simulink library "rappid_564xl_ec_toolbox"  (Simulink 8.1)
settings: Solver=FixedStepDiscrete  StartTime=0.0  StopTime=10.0  RelTol=1e-3
undefined symbols (not defined in the file or in its folder): CTU_unit, mem_AddrLW, mem_AddrUP, rappid_564xl_adc_input_support_rev2, rappid_564xl_can_support_rev2, read_mem_AddrLW, read_mem_AddrUP
(part 1 of 5)
settings Model: Creator=r61406  LastModifiedBy=evarshavskaya

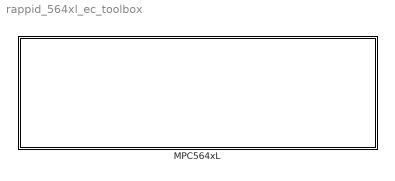
== system rappid_564xl_ec_toolbox ==
  MPC564xL : Subsystem

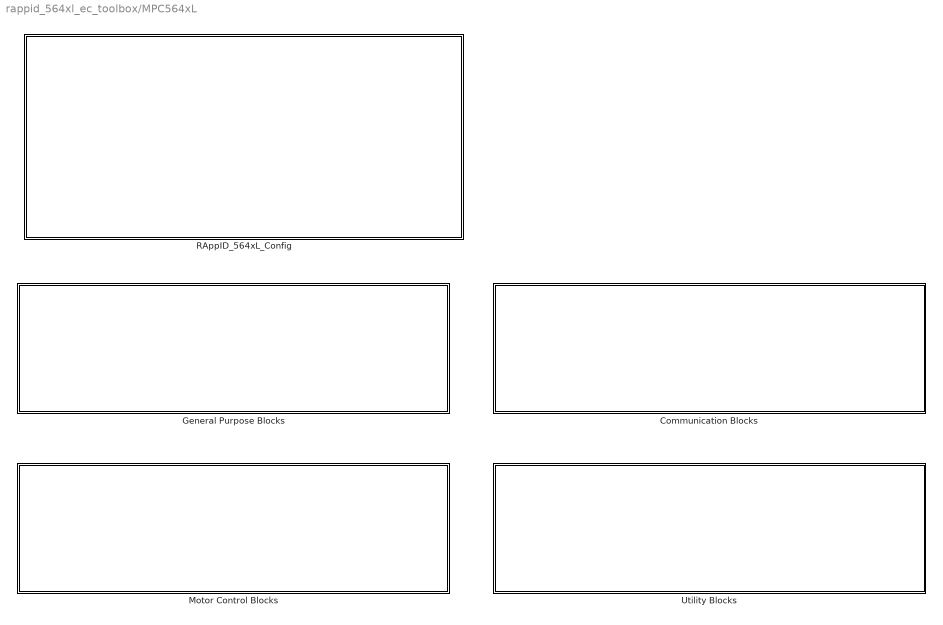
== system rappid_564xl_ec_toolbox/MPC564xL ==
  Communication Blocks : Subsystem
  General Purpose Blocks : Subsystem
  Motor Control Blocks : Subsystem
  RAppID_564xL_Config : Subsystem  LoadFcn=|  InitFcn=|  mask(RAppID_EC_564xL){SystemClock=120, XTAL=40, MC_clock_60=12, MC_clock_80=16, MC_clock_120=10, SWG_clock_60=20, SWG_clock_80=13.334, SWG_clock_120=20, Compiler=CodeWarrior, MemTarget=RAM, Part=MPC5643L, Package=144 LQFP, global_int_priority=11, base_tick_priority=12, sys_task_supress=off, exception_handlers=off, stored_mdl_name=can_simple_block__, freemaster_interface=Oops, freemaster_rx_pin=LINFlex_0 Rx Pin 116 : "PB[3]", freemaster_tx_pin=LINFlex_0 Tx Pin 114 : "PB[2]", freemaster_interface_1=None, freemaster_enable=off, freemaster_rate=57600, freemaster_tx0_pin=18 : B[2] : 114 : A14, freemaster_rx0_pin=19 : B[3] : 116 : B13, freemaster_tx1_pin=57 : D[9] : 26 : L3, freemaster_rx1_pin=29 : B[13] : 60 : R10, freemaster_can_channel=1CH, freemater_can_speed=500K, freemaster_can_msgig=0x7AA, ccp_interface=None, ccp_enable=off, ccp_can_channel=CH1 (MB 0 - 1), ccp_can_speed=500K, ccp_can_cro_id=256, ccp_can_dto_id=257, ccp_dev_id=RappID, ccp_dev_addr=0, ccp_odt=3, ccp_daq=3, pil_enable=off, pil_bam=off, comport=1, pil_rate=57600, bam_password_def=on, bam_password=0xFEEDFACECAFEBEEF, bam_sa_cs=off, bam_start_address=0x0, bam_code_size=0x7000, cons_dspi=on, cons_can=on, cons_adc=on, cons_pwm=on, cons_ctu=on, cons_swg=on, cons_eTimer=on, cons_fm=on}
      | rappid_564xl_set_cur_model(bdroot(gcs));
      | rappid_564xl_block_load(bdroot(gcs)); 
      | rappid_564xl_fmaster_config(gcb);
      | rappid_564xl_set_cur_model(bdroot(gcs));
      | rappid_564xl_update_model('init');
      | rappid_564xl_check('RAppID_EC_564xL');
      | rappid_564xl_consistency_checks( bdroot(gcs));
      mask prompts: SystemClock "Select System Clock Mhz"; XTAL "Select External Crystal Value Mhz"; MC_clock_60 "Motor control clock, MHz  (3.75 - 60)"; MC_clock_80 "Motor control clock, MHz  (5 - 80)"; MC_clock_120 "Motor control clock, MHz  (7.5 - 120)"; SWG_clock_60 "SWG clock, MHz  (12 - 20)"; SWG_clock_80 "SWG clock, MHz  (13.334 - 20)"; SWG_clock_120 "SWG clock, MHz  (12 - 20)"; Compiler "Select Compiler"; MemTarget "Select Target Execution"; Part "Select Part"; Package "Select Package"; global_int_priority "Global Interrupt Priority (0-15)"; base_tick_priority "Base System Tick Priority(0-15)"; sys_task_supress "Suppress System Task"; exception_handlers "Create Exception Handlers"; stored_mdl_name "Stored Model Name"; freemaster_interface "Old Freemaster Interface"; freemaster_rx_pin "Old Rx Pin"; freemaster_tx_pin "Old Tx Pin"; freemaster_interface_1 "Freemaster Interface"; freemaster_enable "Enable Freemaster"; freemaster_rate "Freemaster Interface Rate"; freemaster_tx0_pin "Tx Pin"; freemaster_rx0_pin "Rx Pin"; freemaster_tx1_pin "Tx Pin"; freemaster_rx1_pin "Rx Pin"; freemaster_can_channel "Channel"; freemater_can_speed "Speed"; freemaster_can_msgig "Message ID"; ccp_interface "CCP Interface"; ccp_enable "Enable CCP"; ccp_can_channel "Channel"; ccp_can_speed "Speed"; ccp_can_cro_id "CRO ID (dec value)"; ccp_can_dto_id "DTO ID (dec value)"; ccp_dev_id "DeviceID"; ccp_dev_addr "Device Address (dec value)"; ccp_odt "Max ODT (dec value)"; ccp_daq "Max DAQ (dec value)"; pil_enable "Processor-In-Loop support"; pil_bam "Download Code after build"; comport "COM port number (1,2 ...)"; pil_rate "PIL Baud Rate"; bam_password_def "BAM Default Password"; bam_password "BAM Password"; bam_sa_cs "BAM Manual Start Address and Code Size"; bam_start_address "BAM Start Address"; bam_code_size "BAM Code Size"; cons_dspi "DSPI - Check to enable cross checks; Uncheck to disable cross checks."; cons_can "CAN - Check to enable cross checks; Uncheck to disable cross checks."; cons_adc "ADC - Check to enable cross checks; Uncheck to disable cross checks."; cons_pwm "PWM - Check to enable cross checks; Uncheck to disable cross checks."; cons_ctu "CTU - Check to enable cross checks; Uncheck to disable cross checks."; cons_swg "SWG - Check to enable cross checks; Uncheck to disable cross checks."; cons_eTimer "eTimer - Check to enable cross checks; Uncheck to disable cross checks."; cons_fm "FreeMaster - Check to enable cross checks; Uncheck to disable cross checks."
      mask help: RAppID Toolbox Config block for MPC564xL family of processors.
      mask init:
      | if strcmp(get_param(gcb,'sys_task_supress'),'on')==1,
      |     sysTaskStr = '';
      | else
      |     sysTaskStr = ['System Tick Interrupt Priority : ',get_param(gcb,'base_tick_priority') ,sprintf('\n')];    
      | end
      | 
      | packageStr = get_param(gcb,'Package');
      | 
      | fmaster_interface = get_param(gcb,'freemaster_interface_1');
      | if(strcmp(fmaster_interface,'None')==1)
      |    fmasterStr ='Freemaster : None';
      | else
      |    if((strcmp(fmaster_interface,'Serial 0')==1)||(strcmp(fmaster_interface,'Serial 1')==1))
      |       fmaster_baud_rate = [get_param(gcb,'freemaster_rate'),' Kbits'];
      |     elseif((strcmp(fmaster_interface,'FlexCAN 0')==1)||(strcmp(fmaster_interface,'FlexCAN 1')==1)||(strcmp(fmaster_interface,'FlexCAN2')==1))
      |       fmaster_baud_rate = get_param(gcb,'freemater_can_speed');
      |     end
      |     fmasterStr=['Freemaster : ', fmaster_interface, ' (', fmaster_baud_rate, ')'];
      | end
      | 
      | if (strcmp(get_param(gcb, 'ccp_interface'), 'None')==0)
      |     ccpStr = ['CCP : ', get_param(gcb, 'ccp_interface'), ', 500K'];
      | else
      |     ccpStr = 'CCP : None';
      | end
      | 
      | if strcmp (get_param (gcb, 'pil_enable'), 'on')
      |     comstr = ['Processor-In-Loop : (COM',num2str(get_param (gcb, 'comport')),',',num2str(get_param (gcb, 'pil_rate')),')'];
      | else
      |     if strcmp (get_param (gcb, 'pil_bam'), 'on')
      |         comstr = ['Download Code after build : (COM',num2str(get_param (gcb, 'comport')),')'];
      |     else
      |         comstr = 'Download Code after build : off';
      |     end
      | end
      | maskStr =['System Clock : ', get_param(gcb,'SystemClock'),' MHz',sprintf('\n'),...
      |     'Target : ',get_param(gcb,'Part'), sprintf('\n'),'Package : ',packageStr,sprintf('\n'),...
      |     'XTAL Freq : ',get_param(gcb,'XTAL'),' MHz',sprintf('\n'),...
      |     'Compiler : ', get_param(gcb,'Compiler'), sprintf('\n'),...
      |     'Target Type : ', get_param(gcb,'MemTarget'), sprintf('\n'),...
      |     'Global Interrupt Priority : ',get_param(gcb,'global_int_priority'),sprintf('\n'),...
      |     sysTaskStr,fmasterStr, sprintf('\n'),  ccpStr, sprintf('\n'), comstr];
      settings: CopyFcn=|
      | rappid_564xl_set_cur_model(bdroot(gcs));
      | rappid_564xl_check('RAppID_EC_564xL');
      | rappid_564xl_update_model('copy');
      settings: ModelCloseFcn=|
      | rappid_564xl_set_cur_model(bdroot(gcs));
      | rappid_564xl_model_close;
      settings: NameChangeFcn=|
      | rappid_564xl_model_close;
      | rappid_564xl_change_name;
      settings: CloseFcn=|
      | rappid_564xl_set_cur_model(bdroot(gcs));
      | rappid_564xl_check('RAppID_EC_564xL');
      | rappid_564xl_update_model('copy');
      mask Help: web([rappid_block_help,filesep,'Target_config.htm']);
      mask TypeOptions SystemClock: 60 | 80 | 120
      mask Callback SystemClock:
      | MaskParams = get_param(gcb,'MaskPrompts');
      | MaskEnables = get_param(gcb,'MaskEnables');
      | MaskVis = get_param(gcb, 'MaskVisibilities');
      | 
      | 
      | if (strcmp (get_param (gcb, 'SystemClock'), '120'))
      |     MaskVis{3} = 'off';
      | 	MaskVis{4} = 'off';
      | 	MaskVis{5} = 'on';
      | 
      | 	MaskVis{6} = 'off';
      | 	MaskVis{7} = 'off';
      | 	MaskVis{8} = 'on';
      | elseif (strcmp (get_param (gcb, 'SystemClock'), '80'))
      |     MaskVis{3} = 'off';
      | 	MaskVis{4} = 'on';
      | 	MaskVis{5} = 'off';
      | 
      | 	MaskVis{6} = 'off';
      | 	MaskVis{7} = 'on';
      | 	MaskVis{8} = 'off';
      | elseif (strcmp (get_param (gcb, 'SystemClock'), '60'))
      |     MaskVis{3} = 'on';
      | 	MaskVis{4} = 'off';
      | 	MaskVis{5} = 'off';
      | 
      | 	MaskVis{6} = 'on';
      | 	MaskVis{7} = 'off';
      | 	MaskVis{8} = 'off';
      | end
      | 
      | set_param(gcb,'MaskVisibilities', MaskVis);
      mask TypeOptions XTAL: 8 | 16 | 40
      mask TypeOptions MC_clock_60: 3.75 | 4 | 4.286 | 4.615 | 5 | 5.455 | 6 | 6.667 | 7.5 | 8.571 | 10 | 12 | 15 | 20 | 30 | 60
      mask TypeOptions MC_clock_80: 5 | 5.334 | 5.714 | 6.154 | 6.667 | 7.273 | 8 | 8.889 | 10 | 11.428 | 13.334 | 16 | 20 | 26.667 | 40 | 80
      mask TypeOptions MC_clock_120: 7.5 | 8 | 8.571 | 9.231 | 10 | 10.909 | 12 | 13.334 | 15 | 17.143 | 20 | 24 | 30 | 40 | 60 | 120
      mask TypeOptions SWG_clock_60: 12 | 15 | 20
      mask TypeOptions SWG_clock_80: 13.334 | 16 | 20
      mask TypeOptions SWG_clock_120: 12 | 13.334 | 15 | 17.143 | 20
      mask TypeOptions Compiler: CodeWarrior | Diab | GreenHills
      mask TypeOptions MemTarget: RAM | FLASH
      mask TypeOptions Part: MPC5643L
      mask TypeOptions Package: 144 LQFP | 257 MAPBGA
      mask TypeOptions global_int_priority: 0 | 1 | 2 | 3 | 4 | 5 | 6 | 7 | 8 | 9 | 10 | 11 | 12 | 13 | 14 | 15
      mask TypeOptions base_tick_priority: 0 | 1 | 2 | 3 | 4 | 5 | 6 | 7 | 8 | 9 | 10 | 11 | 12 | 13 | 14 | 15
      mask TypeOptions freemaster_interface: None | Serial | CAN | Oops
      mask TypeOptions freemaster_rx_pin: LINFlex_0 Rx Pin 116 : "PB[3]" | LINFlex_0 Rx Pin 43 : "PB[7]"
      mask TypeOptions freemaster_tx_pin: LINFlex_0 Tx Pin 114 : "PB[2]"
      mask TypeOptions freemaster_interface_1: None | Serial 0 | Serial 1 | FlexCAN 0 | FlexCAN 1
      mask Callback freemaster_interface_1:
      | MaskParams = get_param(gcb,'MaskPrompts');
      | MaskEnables = get_param(gcb,'MaskEnables');
      | MaskVis = get_param(gcb, 'MaskVisibilities');
      | 
      | pos = 1 + length(MaskParams);
      | for i = 1:length(MaskParams)
      |   if strcmp(MaskParams{i}, 'Freemaster Interface Rate')==1
      |     pos = i;
      |     break;
      |   end
      | end
      | 
      | for i = pos:pos+7
      |   MaskVis{i} = 'off';
      | end
      | 
      | if strcmp (get_param (gcb, 'freemaster_interface_1'), 'FlexCAN 0')
      |   set_param(gcb, 'freemaster_enable', 'on');
      |   for i = pos+5:pos+7
      |       MaskVis{i} = 'on';
      |   end
      | end
      | 
      | if strcmp (get_param (gcb, 'freemaster_interface_1'), 'FlexCAN 1')
      |   set_param(gcb, 'freemaster_enable', 'on');
      |   for i = pos+5:pos+7
      |       MaskVis{i} = 'on';
      |   end
      | end
      | 
      | if strcmp (get_param (gcb, 'freemaster_interface_1'), 'Serial 0')
      |   set_param(gcb, 'freemaster_enable', 'on');
      |   MaskVis{pos} = 'on';
      |   for i = pos+1:pos+2
      |     MaskVis{i} = 'on';
      |   end
      | end
      | 
      | if strcmp (get_param (gcb, 'freemaster_interface_1'), 'Serial 1')
      |   set_param(gcb, 'freemaster_enable', 'on');
      |   MaskVis{pos} = 'on';
      |   for i = pos+3:pos+4
      |     MaskVis{i} = 'on';
      |   end
      | end
      | 
      | if strcmp (get_param (gcb, 'freemaster_interface_1'), 'None')
      |   set_param(gcb, 'freemaster_enable', 'off');
      | end
      | 
      | set_param(gcb,'MaskVisibilities', MaskVis);
      | set_param(gcb,'MaskEnables',MaskEnables);
      mask TypeOptions freemaster_rate: 19200 | 38400 | 57600 | 115200 | 230400
      mask TypeOptions freemaster_tx0_pin: 18 : B[2] : 114 : A14
      mask TypeOptions freemaster_rx0_pin: 19 : B[3] : 116 : B13 | 23 : B[7] : 43 : R5
      mask TypeOptions freemaster_tx1_pin: 57 : D[9] : 26 : L3 | 94 : F[14] : 115 : C13
      mask TypeOptions freemaster_rx1_pin: 29 : B[13] : 60 : R10 | 60 : D[12] : 99 : G14 | 95 : F[15] : 113 : D13
      mask TypeOptions freemaster_can_channel: 1CH
      mask TypeOptions freemater_can_speed: 500K
      mask TypeOptions freemaster_can_msgig: 0x7AA
      mask TypeOptions ccp_interface: None | FlexCAN 0 | FlexCAN 1
      mask Callback ccp_interface:
      | MaskParams = get_param(gcb,'MaskPrompts');
      | MaskEnables = get_param(gcb,'MaskEnables');
      | MaskVis = get_param(gcb, 'MaskVisibilities');
      | 
      | pos = 1 + length(MaskParams);
      | for i = 1:length(MaskParams)
      |   if strcmp(MaskParams{i}, 'CCP Interface')==1
      |     pos = i;
      |     break;
      |   end
      | end
      | 
      | for i = pos+2:pos+9
      |   MaskVis{i} = 'off';
      | end
      | 
      | if strcmp (get_param (gcb, 'ccp_interface'), 'None')
      |   set_param(gcb, 'ccp_enable', 'off');
      | else
      |   set_param(gcb, 'ccp_enable', 'on');
      |   for i = pos+2:pos+9
      |       MaskVis{i} = 'on';
      |   end
      | end
      | 
      | set_param(gcb,'MaskVisibilities', MaskVis);
      | set_param(gcb,'MaskEnables',MaskEnables);
      mask TypeOptions ccp_can_channel: CH1 (MB 0 - 1) | CH2 (MB 2 - 3) | CH3 (MB 4 - 5) | CH4 (MB 6 - 7) | CH5 (MB 8 - 9) | CH6 (MB 10 - 11) | CH7 (MB 12 - 13) | CH8 (MB 14 - 15)
      mask TypeOptions ccp_can_speed: 500K
      mask Callback pil_enable:
      | MaskParams = get_param(gcb,'MaskPrompts');
      | MaskEnables = get_param(gcb,'MaskEnables');
      | 
      | for i = 1:length(MaskParams)
      |   if strcmp(MaskParams{i}, 'COM port number (1,2 ...)')==1
      |     top = i;
      |     break;
      |   end
      | end
      | 
      | for i = 1:length(MaskParams)
      |   if strcmp(MaskParams{i}, 'BAM Code Size')==1
      |     bottom = i;
      |     break;
      |   end
      | end
      | 
      | if strcmp (get_param (gcb, 'pil_enable'), 'on')
      |   for i = top:bottom
      |      MaskEnables{i} = 'on';
      |   end
      | else
      |     if (strcmp (get_param (gcb, 'pil_bam'), 'off'))
      |         for i = top:bottom
      |             MaskEnables{i} = 'off';
      |         end
      |     end
      | end
      | 
      | set_param(gcb,'MaskEnables',MaskEnables);
      mask Callback pil_bam:
      | MaskParams = get_param(gcb,'MaskPrompts');
      | MaskEnables = get_param(gcb,'MaskEnables');
      | 
      | for i = 1:length(MaskParams)
      |   if strcmp(MaskParams{i}, 'COM port number (1,2 ...)')==1
      |     top = i;
      |     break;
      |   end
      | end
      | 
      | for i = 1:length(MaskParams)
      |   if strcmp(MaskParams{i}, 'BAM Code Size')==1
      |     bottom = i;
      |     break;
      |   end
      | end
      | 
      | 
      | if ( strcmp (get_param(gcb, 'pil_bam'),'on')   )
      |     for i = top:bottom
      |         MaskEnables{i} = 'on';
      |     end
      | else
      |     if strcmp (get_param(gcb, 'pil_enable'),'off')
      |         for i = top:bottom
      |             MaskEnables{i} = 'off';
      |         end
      |     end
      | end
      | 
      | set_param(gcb,'MaskEnables',MaskEnables);
      mask TypeOptions pil_rate: 19200 | 38400 | 57600 | 115200 | 230400
      mask Callback bam_password_def:
      | maskVis = get_param(gcb, 'MaskVisibilities');
      | MaskParams = get_param(gcb,'MaskPrompts');
      | 
      | pos = 1 + length(MaskParams);
      | for i = 1:length(MaskParams)
      |   if strcmp(MaskParams{i}, 'BAM Password')==1
      |     pos = i;
      |     break;
      |   end
      | end
      | 
      | maskVis{pos} = 'off';
      | if (strcmp(get_param(gcb, 'bam_password_def'), 'off'))
      |     maskVis{pos} = 'on';
      | end
      | 
      | set_param(gcb, 'MaskVisibilities', maskVis);
      mask Callback bam_sa_cs:
      | maskVis = get_param(gcb, 'MaskVisibilities');
      | MaskParams = get_param(gcb,'MaskPrompts');
      | 
      | pos = 1 + length(MaskParams);
      | for i = 1:length(MaskParams)
      |   if strcmp(MaskParams{i}, 'BAM Start Address')==1
      |     pos = i;
      |     break;
      |   end
      | end
      | 
      | maskVis{pos} = 'off';
      | maskVis{pos+1} = 'off';
      | if (strcmp(get_param(gcb, 'bam_sa_cs'), 'on'))
      |     maskVis{pos} = 'on';
      |     maskVis{pos+1} = 'on';
      | end
      | 
      | set_param(gcb, 'MaskVisibilities', maskVis);
      mask Display:
      | text(0.01,0.95,'RAppID MPC564xL Target Setup');
      | disp(maskStr);
  Utility Blocks : Subsystem
